simulink model "ME131_lab8"  (R2018b)
settings: Solver=ode15s  StartTime=0.0  StopTime=29  MinStep=1e-100  RelTol=1e-3
values from neighbouring files (symbols this model uses):
  Cf = 48703    [ME131_lab_main.m]
  Cr = 57269    [ME131_lab_main.m]
  dt = 0.001    [ME131_lab_main.m]
  Iz = 3477    [ME131_lab_main.m]
  Lf = 1.15214    [ME131_lab_main.m]
  Lr = 1.69286    [ME131_lab_main.m]
  m = 1830.59    [ME131_lab_main.m]
  Vx0 = 11.901    [ME131_lab_main.m]
  Vy0 = 0    [ME131_lab_main.m]
  X0 = 49.41    [ME131_lab_main.m]
  Y0 = 49.33807    [ME131_lab_main.m]
  yaw0 = 3.930132    [ME131_lab_main.m]
  yawRate0 = 0    [ME131_lab_main.m]
settings Model: Creator=YW_Liao  LastModifiedBy=Sunny
settings SFSimCC: SimUseLocalCustomCode=off
settings RTWCC: RTWUseLocalCustomCode=off

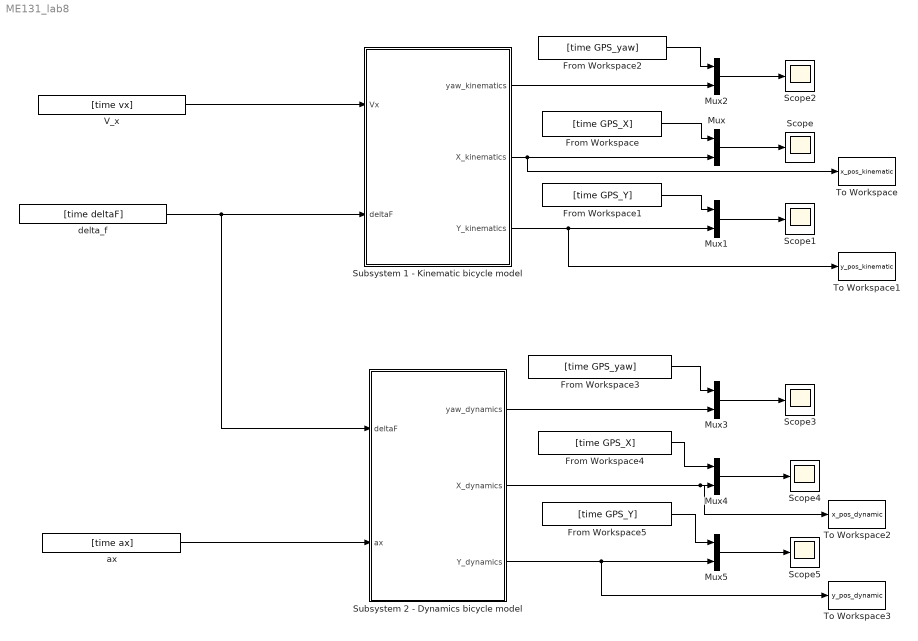
== system ME131_lab8 ==
  From Workspace : FromWorkspace  VariableName=[time GPS_X]  SampleTime=dt
  From Workspace1 : FromWorkspace  VariableName=[time GPS_Y]  SampleTime=dt
  From Workspace2 : FromWorkspace  VariableName=[time GPS_yaw]  SampleTime=dt
  From Workspace3 : FromWorkspace  VariableName=[time GPS_yaw]  SampleTime=dt
  From Workspace4 : FromWorkspace  VariableName=[time GPS_X]  SampleTime=dt
  From Workspace5 : FromWorkspace  VariableName=[time GPS_Y]  SampleTime=dt
  Mux{,1..5} (6 alike) : Mux  Inputs=2
  Scope{,1..5} (6 alike) : Scope
  Subsystem 1 - Kinematic bicycle model : Subsystem
  Subsystem 2 - Dynamics bicycle model : Subsystem
  To Workspace : ToWorkspace  VariableName=x_pos_kinematic  SaveFormat=Timeseries  SampleTime=-1
  To Workspace1 : ToWorkspace  VariableName=y_pos_kinematic  SaveFormat=Timeseries  SampleTime=-1
  To Workspace2 : ToWorkspace  VariableName=x_pos_dynamic  SaveFormat=Timeseries  SampleTime=-1
  To Workspace3 : ToWorkspace  VariableName=y_pos_dynamic  SaveFormat=Timeseries  SampleTime=-1
  V_x : FromWorkspace  VariableName=[time vx]  SampleTime=dt
  ax : FromWorkspace  VariableName=[time ax]  SampleTime=dt
  delta_f : FromWorkspace  VariableName=[time deltaF]  SampleTime=dt
  wires:
  Mux1/1 -> Scope1/1
  Mux/1 -> Scope/1
  From Workspace/1 -> Mux/1
  From Workspace1/1 -> Mux1/1
  Mux2/1 -> Scope2/1
  From Workspace2/1 -> Mux2/1
  From Workspace4/1 -> Mux4/1
  From Workspace3/1 -> Mux3/1
  Mux3/1 -> Scope3/1
  Mux4/1 -> Scope4/1
  Mux5/1 -> Scope5/1
  From Workspace5/1 -> Mux5/1
  Subsystem 1 - Kinematic bicycle model/3(Y_kinematics) -> To Workspace1/1, Mux1/2
  Subsystem 1 - Kinematic bicycle model/2(X_kinematics) -> To Workspace/1, Mux/2
  V_x/1 -> Subsystem 1 - Kinematic bicycle model/1(Vx)
  delta_f/1 -> Subsystem 1 - Kinematic bicycle model/2(deltaF), Subsystem 2 - Dynamics bicycle model/1(deltaF)
  Subsystem 1 - Kinematic bicycle model/1(yaw_kinematics) -> Mux2/2
  ax/1 -> Subsystem 2 - Dynamics bicycle model/2(ax)
  Subsystem 2 - Dynamics bicycle model/1(yaw_dynamics) -> Mux3/2
  Subsystem 2 - Dynamics bicycle model/2(X_dynamics) -> To Workspace2/1, Mux4/2
  Subsystem 2 - Dynamics bicycle model/3(Y_dynamics) -> To Workspace3/1, Mux5/2

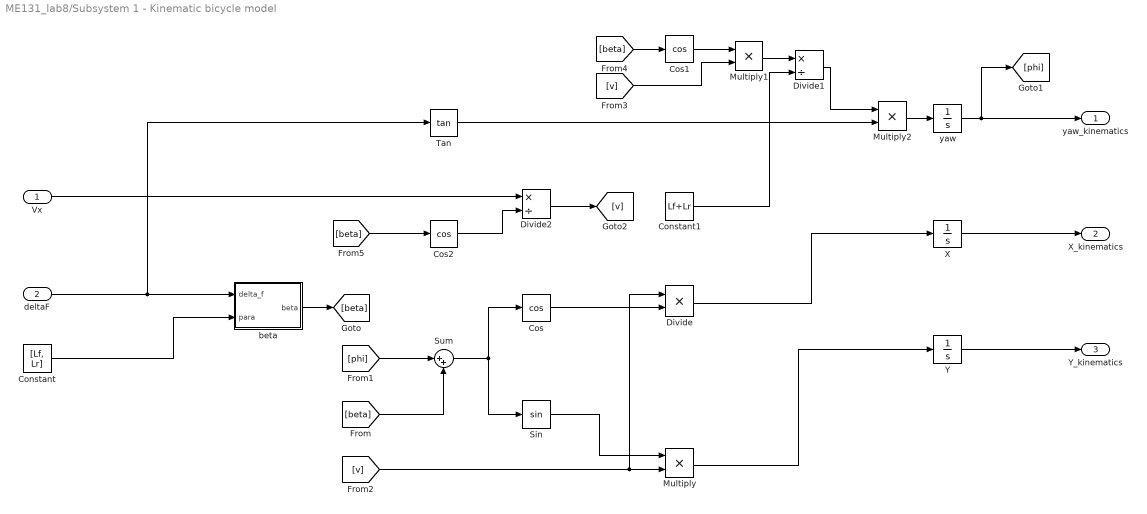
== system ME131_lab8/Subsystem 1 - Kinematic bicycle model ==
  Vx : Inport
  deltaF : Inport  Port=2
  Constant : Constant  Value=[Lf, Lr]
  Constant1 : Constant  Value=Lf+Lr
  Cos : Trigonometry  Operator=cos
  Cos1 : Trigonometry  Operator=cos
  Cos2 : Trigonometry  Operator=cos
  Divide : Product  Inputs=**
  Divide1 : Product  Inputs=*/
  Divide2 : Product  Inputs=*/
  Multiply : Product
  Multiply1 : Product
  Multiply2 : Product
  Sin : Trigonometry
  Sum : Sum  Inputs=|++
  Tan : Trigonometry  Operator=tan
  X : Integrator  InitialCondition=X0
  Y : Integrator  InitialCondition=Y0
  beta : MATLAB Function  TreatAsAtomicUnit=on
  yaw : Integrator  InitialCondition=yaw0
  yaw_kinematics : Outport
  X_kinematics : Outport  Port=2
  Y_kinematics : Outport  Port=3
  wires:
  X/1 -> X_kinematics/1
  Y/1 -> Y_kinematics/1
  Constant/1 -> beta/2(para)
  beta/1(beta) -> [beta]
  [phi] -> Sum/1
  [beta] -> Sum/2
  Sum/1 -> Sin/1, Cos/1
  Cos/1 -> Divide/2
  [v] -> Divide/1, Multiply/2
  Multiply/1 -> Y/1
  [beta] -> Cos1/1
  Cos1/1 -> Multiply1/1
  [v] -> Multiply1/2
  Multiply1/1 -> Divide1/1
  Sin/1 -> Multiply/1
  deltaF/1 -> Tan/1, beta/1(delta_f)
  Divide1/1 -> Multiply2/1
  Multiply2/1 -> yaw/1
  Tan/1 -> Multiply2/2
  Constant1/1 -> Divide1/2
  [beta] -> Cos2/1
  Cos2/1 -> Divide2/2
  Divide2/1 -> [v]
  Divide/1 -> X/1
  Vx/1 -> Divide2/1
  yaw/1 -> yaw_kinematics/1, [phi]

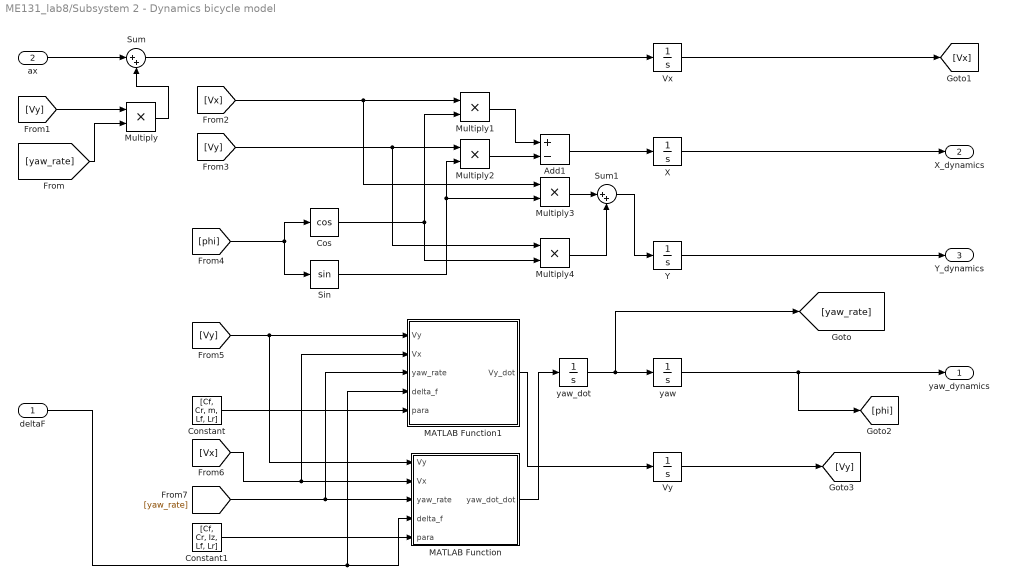
== system ME131_lab8/Subsystem 2 - Dynamics bicycle model ==
  deltaF : Inport
  ax : Inport  Port=2
  Add1 : Sum  Inputs=+-
  Constant : Constant  Value=[Cf, Cr, m, Lf, Lr]
  Constant1 : Constant  Value=[Cf, Cr, Iz, Lf, Lr]
  Cos : Trigonometry  Operator=cos
  MATLAB Function : MATLAB Function  TreatAsAtomicUnit=on
  MATLAB Function1 : MATLAB Function  TreatAsAtomicUnit=on
  Multiply{,1..4} (5 alike) : Product
  Sin : Trigonometry
  Sum : Sum  Inputs=|++
  Sum1 : Sum  Inputs=|++
  Vx : Integrator  InitialCondition=Vx0
  Vy : Integrator  InitialCondition=Vy0
  X : Integrator  InitialCondition=X0
  Y : Integrator  InitialCondition=Y0
  yaw : Integrator  InitialCondition=yaw0
  yaw_dot : Integrator  InitialCondition=yawRate0
  yaw_dynamics : Outport
  X_dynamics : Outport  Port=2
  Y_dynamics : Outport  Port=3
  wires:
  Y/1 -> Y_dynamics/1
  yaw_dot/1 -> [yaw_rate], yaw/1
  X/1 -> X_dynamics/1
  yaw/1 -> [phi], yaw_dynamics/1
  deltaF/1 -> MATLAB Function/4(delta_f), MATLAB Function1/4(delta_f)
  ax/1 -> Sum/1
  [Vy] -> Multiply/1
  [yaw_rate] -> Multiply/2
  Multiply/1 -> Sum/2
  Sum/1 -> Vx/1
  Vx/1 -> [Vx]
  [phi] -> Sin/1, Cos/1
  [Vx] -> Multiply3/1, Multiply1/1
  Cos/1 -> Multiply1/2, Multiply4/2
  [Vy] -> Multiply2/1, Multiply4/1
  Sin/1 -> Multiply3/2, Multiply2/2
  Multiply1/1 -> Add1/1
  Multiply2/1 -> Add1/2
  Add1/1 -> X/1
  Multiply3/1 -> Sum1/1
  Multiply4/1 -> Sum1/2
  Sum1/1 -> Y/1
  [Vy] -> MATLAB Function/1(Vy), MATLAB Function1/1(Vy)
  [Vx] -> MATLAB Function1/2(Vx), MATLAB Function/2(Vx)
  [yaw_rate] -> MATLAB Function/3(yaw_rate), MATLAB Function1/3(yaw_rate)
  Vy/1 -> [Vy]
  Constant/1 -> MATLAB Function1/5(para)
  Constant1/1 -> MATLAB Function/5(para)
  MATLAB Function/1(yaw_dot_dot) -> yaw_dot/1
  MATLAB Function1/1(Vy_dot) -> Vy/1

== matlab function ME131_lab8/Subsystem 1 - Kinematic bicycle model/beta ==
  data: delta_f input; beta output; para input
function beta = fcn(delta_f, para)
lr = para(2);
lf = para(1);
beta = atan(lr/(lr+lf)*tan(delta_f));
end

== matlab function ME131_lab8/Subsystem 2 - Dynamics bicycle model/MATLAB Function ==
  data: Vy input; yaw_dot_dot output; Vx input; yaw_rate input; delta_f input; para input
function yaw_dot_dot = fcn(Vy,Vx,yaw_rate,delta_f,para)
Cf = para(1);
Cr = para(2);
Iz = para(3);
Lf = para(4);
Lr = para(5);

yaw_dot_dot = Lf*Cf/Iz*(delta_f - (Vy+Lf*yaw_rate)/Vx)...
     - Lr*Cr/Iz*(-Vy+Lr*yaw_rate)/Vx;
end

== matlab function ME131_lab8/Subsystem 2 - Dynamics bicycle model/MATLAB Function1 ==
  data: Vy input; Vy_dot output; Vx input; yaw_rate input; delta_f input; para input
function  Vy_dot = fcn(Vy, Vx, yaw_rate,delta_f,para)
Cf = para(1);
Cr = para(2);
m = para(3);
Lf = para(4);
Lr = para(5);
Vy_dot = Cf/m*(delta_f - (Vy+Lf*yaw_rate)/Vx)...
    +Cr/m*(-Vy+Lr*yaw_rate)/Vx - yaw_rate*Vx;
